simulink model "ex1"  (R2020a)
settings: Solver=VariableStepAuto  StartTime=0.0  StopTime=10.0  RelTol=1e-3
settings Model: Creator=EREN  LastModifiedBy=EREN

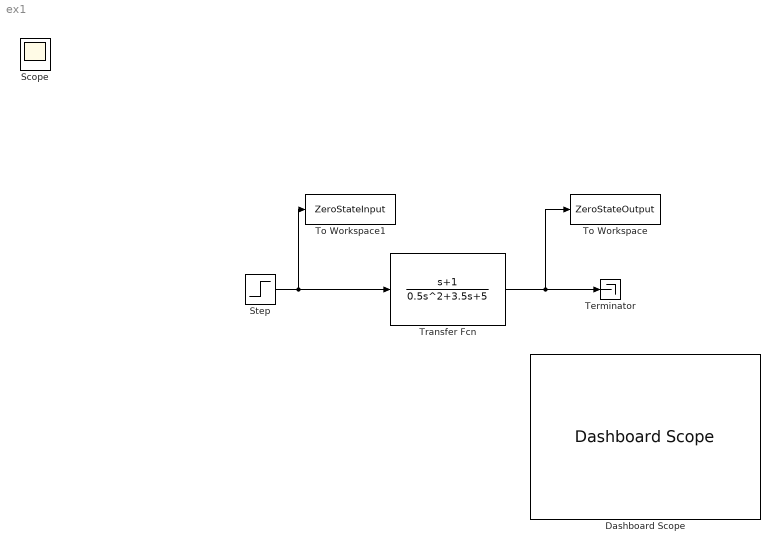
== system ex1 ==
  Dashboard Scope : DashboardScope
  Step : Step  After=100  SampleTime=0
  Terminator : Terminator
  To Workspace : ToWorkspace  VariableName=ZeroStateOutput  SaveFormat=Timeseries  SampleTime=-1
  To Workspace1 : ToWorkspace  VariableName=ZeroStateInput  SaveFormat=Timeseries  SampleTime=-1
  Transfer Fcn : TransferFcn  Numerator=[1 1]  Denominator=[0.5 3.5 5]
  Scope : Scope
  wires:
  Transfer Fcn/1 -> Terminator/1, To Workspace/1
  Step/1 -> Transfer Fcn/1, To Workspace1/1
